simulink model "testStateflow"  (R2014a)
settings: Solver=FixedStepDiscrete  StartTime=0.0  StopTime=Inf  FixedStep=0.001  RelTol=1e-3
settings Model: BufferReuse=off  Creator=djoshea  LastModifiedBy=djoshea
settings SolverCC: EnableConcurrentExecution=on
settings OptimizationCC: BlockReduction=off  OptimizeBlockIOStorage=off  BufferReuse=off  GlobalBufferReuse=off  ExpressionFolding=off  LocalBlockOutputs=off
settings HardwareCC: ProdIntDivRoundTo=Zero  ProdEndianess=LittleEndian  ProdHWDeviceType=Generic->32-bit x86 compatible
settings RTWCC: SystemTargetFile=slrt.tlc  TemplateMakefile=slrt_default_tmf  Description=Simulink Real-Time  ProcessScript=slrt_make_rtw_hook  RTWCompilerOptimization=On
settings SimulinkRealTimeCC: GeneratePreprocessorConditionals=Disable all  EnableShiftOperators=on

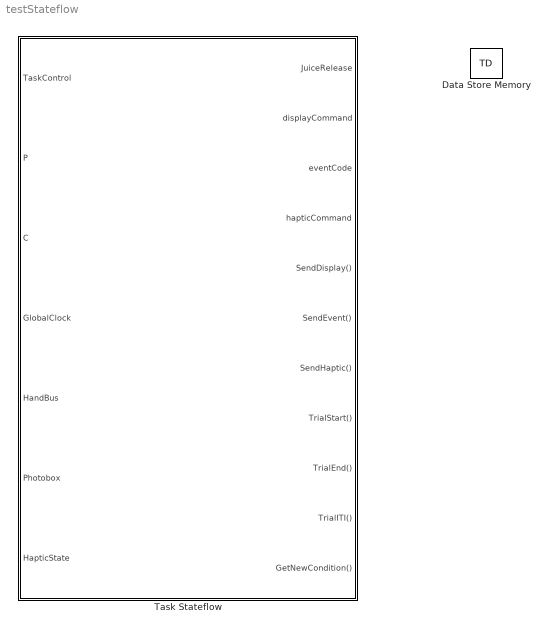
== system testStateflow ==
  Data Store Memory : DataStoreMemory  DataStoreName=TD  ReadBeforeWriteMsg=warning  WriteAfterWriteMsg=warning  WriteAfterReadMsg=warning  OutDataTypeStr=Bus: TrialDataBus
  Task Stateflow : Stateflow chart  TreatAsAtomicUnit=on

== stateflow chart testStateflow/Task Stateflow ==
  state TaskControl [parallel]
    settings: executionOrder=1
    state Task
      state TaskFlow [parallel]
        ex:
        send(HapticReset, HapticMoveHoldControl);
        send(HapticDisallowPerturbation, HapticPerturbationControl);
        send(AbortJuice, JuiceToggle);
        settings: executionOrder=1
        state InitTrial
          en:
          send(TrialStart);
          TD.taskRunning = uint8(1);
          displayCommand = DisplayCommand.InitTrial;
          send(SendDisplay);
          hapticCommand = HapticCommand.SupportAtCenter;
          send(SendHaptic);
          send(HapticAllowPerturbation, HapticPerturbationControl);
          eventCode = TaskEvent.CenterOnset;
          state = TaskState.InitTrial;
          TD.timeInitTrial = GlobalClock;
          TD.timeGoCueCommand = uint32(0);
          TD.timeGoCue = uint32(0);
          TD.timeTargetOnsetCommand = uint32(0);
          TD.timeTargetOnset = uint32(0);
          TD.timeMove = uint32(0);
          TD.rt = uint32(0);
          TD.rtNominal = uint32(0);
          TD.delay = uint32(0);
          TD.iti = uint32(0);
          TD.holdXCenter = 0;
          TD.holdYCenter = 0;
          TD.holdXTarget = 0;
          TD.holdYTarget = 0;
          TD.targetXCurrent = 0;
          TD.targetYCurrent = 0;
          TD.targetWidthCurrent = 0;
          TD.targetDepthCurrent = 0;
          TD.hapticPerturbationOccurred = uint8(0);
          TD.hitObstacleThisTrial = uint8(0);
          TD.consecutiveNoStarts = TD.consecutiveNoStarts + uint16(1);
          TD.isTouchingTarget = uint8(0);
          TD.hasMissedTarget = uint8(0);
          TD.substantiveFailure = uint8(0);
          TD.moveOnsetThreshOccurred = uint8(0);
        state CenterAcquireHold
          state CenterAcquireLogic [parallel]
            settings: executionOrder=1
            state WaitCenterSettle
              en:
              state = TaskState.WaitCenterSettle;
              displayCommand = DisplayCommand.CenterAcquired;
              send(SendDisplay);
              eventCode = TaskEvent.CenterAcquired;
              send(SendEvent);
              ex:
              % Establish hold window for td.isHolding
              TD.holdXCenter = HandBus.handX;
              TD.holdYCenter = HandBus.handY;
            state WaitCenterAcquire
              en:
              state = TaskState.WaitCenterAcquire;
              displayCommand = DisplayCommand.CenterOnset;
              send(SendDisplay);
              eventCode = TaskEvent.CenterOnset;
              send(SendEvent);
              % Move the hand to the center (while he's holding on)
              send(HapticMoveToCenter, HapticMoveHoldControl);
            state WaitCenterHold
              en:
              state = TaskState.WaitCenterHold;
              displayCommand = DisplayCommand.CenterSettled;
              send(SendDisplay);
              eventCode = TaskEvent.CenterSettled;
              send(SendEvent);
              % Either stop moving to center or hold the haptic for the delay period
              send(HapticArrivedAtCenter, HapticMoveHoldControl);
            state CenterUnacquire
              en:
              displayCommand = DisplayCommand.CenterUnacquire;
              send(SendDisplay);
              eventCode = TaskEvent.CenterUnacquire;
              send(SendEvent);
            state CenterHeld
              en:
              displayCommand = DisplayCommand.CenterHeld;
              send(SendDisplay);
              eventCode = TaskEvent.CenterHeld;
              send(SendEvent);
              % always send target to haptic, command packet will indicate
              % whether viscosity is needed
              hapticCommand = HapticCommand.CreateTarget;
              send(SendHaptic);
              if P.timeJuiceCenter > 0
              TD.juiceNumDrops = uint16(1);
              TD.juiceDropSize = uint16(P.timeJuiceCenter);
              send(SendJuice, JuiceToggle);
              end
            WaitCenterAcquire -> WaitCenterSettle [order 1] : [TD.isTouchingCenter == 1]
            CenterUnacquire -> WaitCenterAcquire
            WaitCenterSettle -> WaitCenterHold : after(P.timeCenterSettle,tick)
                | % Wait for settling before enforcing hold
            WaitCenterHold -> CenterUnacquire [order 3] : [~TD.isHoldingCenter && P.allowReacquireCenter]
                | % Moved during center hold --> allow re-aquire
            WaitCenterHold -> CenterHeld [order 2] : after(P.timeCenterHold,tick)
                | % Held center
        state StartTask
          en:
          state = TaskState.StartTask;
          displayCommand = DisplayCommand.StartTask;
          send(SendDisplay);
        state GetNewTrialParams
          en:
          send(GetNewCondition);
        state HoldingHaptic
          state DelayPeriodGoCue
            state ShowObstacle
              en:
              hapticCommand = HapticCommand.CreateGap;
              send(SendHaptic);
              displayCommand = DisplayCommand.ObstacleOnset;
              send(SendDisplay);
              eventCode = TaskEvent.ObstacleOnset;
              send(SendEvent);
            state GoCue
              en:
              send(HapticGoCue, HapticMoveHoldControl);
              state GoCueZeroDelay
                en:
                state = TaskState.GoCueZeroDelay;
                TD.timeGoCueCommand = GlobalClock;
                displayCommand = DisplayCommand.GoCueZeroDelay;
                send(SendDisplay);
                eventCode = TaskEvent.TargetOnsetCommand;
                send(SendEvent);
                eventCode = TaskEvent.GoCueCommand;
                send(SendEvent);
              state GoCueNonZeroDelay
                en:
                state = TaskState.GoCueNonZeroDelay;
                TD.timeGoCueCommand = GlobalClock;
                displayCommand = DisplayCommand.GoCueNonZeroDelay;
                send(SendDisplay);
                eventCode = TaskEvent.GoCueCommand;
                send(SendEvent);
            state SetTargetInfo
              en:
              TD.targetXCurrent = C.targetX;
              TD.targetYCurrent = C.targetY;
              TD.targetWidthCurrent = C.targetWidth;
              TD.targetDepthCurrent = C.targetDepth;
            state DelayPeriod
              en:
              state = TaskState.DelayPeriod;
              TD.timeTargetOnsetCommand = GlobalClock;
              displayCommand = DisplayCommand.DelayPeriodStart;
              send(SendDisplay);
              eventCode = TaskEvent.TargetOnsetCommand;
              send(SendEvent);
            state WaitMoveOnset
              en:
              state = TaskState.WaitMoveOnset;
              du:
              TD.rt = GlobalClock - TD.timeGoCue; % detected by photobox
              TD.rtNominal = GlobalClock - TD.timeGoCueCommand; % not detected by photobox
              ex:
              TD.timeMove = GlobalClock;
              TD.rt = GlobalClock - TD.timeGoCue; % not detected by photobox
              TD.rtNominal = GlobalClock - TD.timeGoCueCommand; % not detected by photobox
              send(HapticMoveOnset, HapticMoveHoldControl);
              displayCommand = DisplayCommand.MoveOnset;
              send(SendDisplay)
              eventCode = TaskEvent.MoveOnsetOnline;
              send(SendEvent);
            (default) -> (junction 1909)
            (junction 1909) -> ShowObstacle [order 1] : [C.hasChannel]
            (junction 1909) -> SetTargetInfo [order 2]
            ShowObstacle -> (junction 1923) [order 2] : [~TD.isHoldingCenter]
                | % Moved during delay
            ShowObstacle -> SetTargetInfo [order 1] : % Show obstacle first, then target
                | after(C.timeObstacleOnsetBeforeTarget, tick)
            SetTargetInfo -> GoCueZeroDelay [order 1] : [C.delayNominal == 0]
                | % Zero Delay
            DelayPeriod -> (junction 1923) [order 1] : [~TD.isHoldingCenter]
                | % Moved during delay
            SetTargetInfo -> DelayPeriod [order 2] : % Non-zero Delay
            DelayPeriod -> GoCueNonZeroDelay [order 2] : after(C.delayNominal, tick)
                | % Delay period over
            GoCue -> WaitMoveOnset : after(1,tick)
            WaitMoveOnset -> (junction 1269) [order 2] : [~TD.isHoldingCenter]
                | % Move from center
          state TargetAcquireHold
            state WaitTargetAcquire
              en:
              TD.consecutiveNoStarts = uint16(0); % count as initiated the trial
              state = TaskState.WaitTargetAcquire;
            state WaitTargetHold
              en:
              send(HapticHoldAtTarget, HapticMoveHoldControl);
              TD.holdXTarget = HandBus.handX;
              TD.holdYTarget = HandBus.handY;
              state = TaskState.WaitTargetHold;
              displayCommand = DisplayCommand.TargetSettled;
              send(SendDisplay);
              eventCode = TaskEvent.TargetSettled;
              send(SendEvent);
              ex:
              displayCommand = DisplayCommand.TargetHeld;
              send(SendDisplay);
              eventCode = TaskEvent.TargetHeld;
              send(SendEvent);
            WaitTargetAcquire -> WaitTargetHold [order 2] : [TD.isTouchingTarget || currentlyTouching]
                | % Target Acquired
          (junction 1269) -> WaitTargetAcquire [order 1] : [TD.rtNominal >= P.rtMin]
              | % RT acceptable
        state TrialFailure
          en:
          TD.success = uint8(0);
          send(HapticDisallowPerturbation, HapticPerturbationControl);
          state FailureCenterAcquire
            en:
            TD.substantiveFailure = uint8(0);
            state = TaskState.FailureCenterAcquire;
            TD.getNewTrialParams = uint8(0);
            displayCommand = DisplayCommand.FailureCenterFlyAway;
            send(SendDisplay);
            eventCode = TaskEvent.FailureToAcquireCenter;
            send(SendEvent);
          state FailureComputeITI
            en:
            if P.repeatUntilSuccess
            TD.getNewTrialParams = uint8(0);
            end
            TD.failureCode = state;
            computeFailureITI();
          state FailureHitObstacle
            en:
            state = TaskState.FailureHitObstacle;
            TD.getNewTrialParams = uint8(1);
            TD.substantiveFailure = uint8(1);
            displayCommand = DisplayCommand.FailureHitObstacle;
            send(SendDisplay);
            eventCode = TaskEvent.FailureHitObstacle;
            send(SendEvent);
          state FailureClearObstacles
            en:
            hapticCommand = HapticCommand.ClearObstacles;
            send(SendHaptic);
          state FailureCenterHold
            en:
            TD.substantiveFailure = uint8(0);
            state = TaskState.FailureCenterHold;
            TD.getNewTrialParams = uint8(0);
            displayCommand = DisplayCommand.FailureCenterFlyAway;
            send(SendDisplay);
            eventCode = TaskEvent.FailureBrokeCenterHold;
            send(SendEvent);
          state FailureDelayMove
            en:
            TD.substantiveFailure = uint8(0);
            state = TaskState.FailureDelayMove;
            TD.getNewTrialParams = uint8(1);
            displayCommand = DisplayCommand.FailureTargetFlyAway;
            send(SendDisplay);
            eventCode = TaskEvent.FailureBrokeCenterHoldDelay;
            send(SendEvent);
          state FailureRTTooFast
            en:
            TD.substantiveFailure = uint8(0);
            state = TaskState.FailureRTTooFast;
            TD.getNewTrialParams = uint8(0);
            displayCommand = DisplayCommand.FailureTargetFlyAway;
            send(SendDisplay);
            eventCode = TaskEvent.FailureRTTooFast;
            send(SendEvent);
          state FailureRTTooSlow
            en:
            TD.substantiveFailure = uint8(0);
            state = TaskState.FailureRTTooSlow;
            TD.getNewTrialParams = uint8(0);
            displayCommand = DisplayCommand.FailureTargetFlyAway;
            send(SendDisplay);
            eventCode = TaskEvent.FailureRTTooSlow;
            send(SendEvent);
          state FailureMissedTarget
            en:
            TD.substantiveFailure = uint8(1);
            state = TaskState.FailureTargetMissed;
            TD.getNewTrialParams = uint8(1);
            displayCommand = DisplayCommand.FailureTargetFlyAway;
            send(SendDisplay);
            eventCode = TaskEvent.MissedTarget;
            send(SendEvent);
            eventCode = TaskEvent.FailureTargetMissed;
            send(SendEvent);
          state FailureTargetAcquire
            en:
            TD.substantiveFailure = uint8(1);
            state = TaskState.FailureTargetAcquire;
            TD.getNewTrialParams = uint8(1);
            displayCommand = DisplayCommand.FailureTargetFlyAway;
            send(SendDisplay);
            eventCode = TaskEvent.FailureToAcquireTarget;
            send(SendEvent);
          state FailureHapticReleased
            en:
            TD.substantiveFailure = uint8(0);
            state = TaskState.FailureHapticReleased;
            TD.getNewTrialParams = uint8(1);
            displayCommand = DisplayCommand.FailureTargetFlyAway;
            send(SendDisplay);
            eventCode = TaskEvent.FailureHapticReleased;
            send(SendEvent);
          FailureCenterAcquire -> (junction 1353)
          FailureHitObstacle -> (junction 1857) : % Bypass obstacle clearing when hit
          (junction 1857) -> FailureComputeITI
          FailureClearObstacles -> (junction 1857)
          (junction 1353) -> FailureClearObstacles : after(1,tick)
          FailureCenterHold -> (junction 1353)
          FailureHapticReleased -> (junction 1353)
          FailureDelayMove -> (junction 1353)
          FailureRTTooFast -> (junction 1353)
          FailureTargetAcquire -> (junction 1353)
          FailureRTTooSlow -> (junction 1353)
          FailureMissedTarget -> (junction 1353)
        state ITI
          en:
          send(TrialEnd);
          state = TaskState.ITI;
          displayCommand = DisplayCommand.ITI;
          send(SendDisplay);
          send(TrialITI);
          % Reset the haptic to normal state
          send(HapticReset, HapticMoveHoldControl);
          send(HapticDisallowPerturbation, HapticPerturbationControl);
        state Success
          en:
          state = TaskState.Success;
          TD.success = uint8(1);
          TD.getNewTrialParams = uint8(1);
          computeRewardAndITI();
          send(SendJuice, JuiceToggle);
          displayCommand = DisplayCommand .Success;
          send(SendDisplay);
          eventCode = TaskEvent.Success;
          send(SendEvent);
        (default) -> StartTask
        GetNewTrialParams -> InitTrial : after(1, tick)
        (junction 1387) -> InitTrial [order 2] : % Re-use the old trial params
        StartTask -> GetNewTrialParams : after(1,tick)
        (junction 1387) -> GetNewTrialParams [order 1] : [TD.getNewTrialParams>0]
            | % New condition needed
        ITI -> (junction 1387) : after(TD.iti,tick)
            | % Wait ITI
        Success -> ITI : after(P.timeRewardFeedback,tick)
            | % Wait for target white flash
        WaitTargetAcquire -> FailureMissedTarget [order 3] : % Went past planar stop target
            | [TD.hasMissedTarget && P.failOnMissedTarget]
        FailureComputeITI -> ITI : after(TD.timeFailureFeedback,tick)
        WaitCenterAcquire -> FailureCenterAcquire [order 2] : after(P.timeCenterAcquire,tick)
            | % Did not acquire center
        WaitCenterHold -> FailureCenterHold [order 1] : [~TD.isHoldingCenter && ~P.allowReacquireCenter]
            | % Moved during center hold --> fail trial
        (junction 1923) -> CenterUnacquire [order 2] : [P.allowReacquireCenter]
            | % Moved during delay --> allow-reacquire
        WaitTargetAcquire -> FailureTargetAcquire [order 1] : after(P.timeTargetAcquire, tick)
            | % Did not acquire target
        InitTrial -> WaitCenterAcquire : after(1,tick)
        (junction 1923) -> FailureDelayMove [order 1] : [~P.allowReacquireCenter]
            | % Moved during delay -> fail trial
        CenterHeld -> DelayPeriodGoCue
        WaitTargetHold -> Success : after(P.timeTargetHold, tick)
            | % Held target
        HoldingHaptic -> FailureHitObstacle [order 2] : [HapticState.hitObstacle && ...
            | (~C.obstacleCollisionPermitted)]
            | % Hit red obstacle
        (junction 1269) -> FailureRTTooFast [order 2] : [TD.rtNominal < P.rtMin]
            | % RT too fast
        WaitMoveOnset -> FailureRTTooSlow [order 1] : after(P.rtMax,tick)
            | % RT too slow
        HoldingHaptic -> FailureHapticReleased [order 1] : [~HandBus.handSeen]
            | % Released haptic device
      state HapticObstacleState [parallel]
        settings: executionOrder=6
        state DebounceRelease
        state NotColliding
        state DebounceHit
        state Colliding
          en:
          TD.hitObstacleThisTrial = uint8(1);
          displayCommand = DisplayCommand.HitObstacle;
          send(SendDisplay);
          eventCode = TaskEvent.HitObstacle;
          send(SendEvent);
          ex:
          displayCommand = DisplayCommand.ReleasedObstacle;
          send(SendDisplay);
          eventCode = TaskEvent.ReleasedObstacle;
          send(SendEvent);
        (default) -> NotColliding
        DebounceRelease -> DebounceHit [order 1] : [HapticState.hitObstacle == 1]
        DebounceRelease -> NotColliding [order 2] : after(100, tick)
        DebounceHit -> DebounceRelease : [HapticState.hitObstacle==0]
        Colliding -> DebounceRelease : [HapticState.hitObstacle==0]
        NotColliding -> Colliding : [HapticState.hitObstacle == 1]
      state ComputeHandState [parallel]
        en,du:
        if state ~= TaskState.InitTrial
        % determine if we're within the center hold windows
        TD.isTouchingCenter = isTouching(C.centerX, C.centerY, P.centerSize);
        TD.isHoldingCenter = uint8(isTouching(TD.holdXCenter, TD.holdYCenter, P.holdWindowCenter) && ~HandBus.handMoving);
        % always use haptic coordinates to determine touching
        % if hand passes vertically above target without colliding, register a miss
        currentlyTouching = uint8(0);
        currentlyPastTarget = uint8(0);
        [currentlyTouching, currentlyPastTarget] = isTouchingBarTarget();
        if ~TD.hasMissedTarget && currentlyTouching && TD.timeTargetOnsetCommand > 0
        % mark target as touched
        TD.isTouchingTarget = uint8(1);
        end
        if ~TD.isTouchingTarget && ~TD.hasMissedTarget && currentlyPastTarget && TD.timeTargetOnsetCommand > 0
        % mark target as missed
        TD.hasMissedTarget = uint8(1);
        end
        if TD.timeGoCueCommand > 0
        % figure out our distance/velocity in direction of target
        [TD.distanceTowardsTarget, TD.velocityTowardsTarget] = computeProgressTowardsTarget();
        if ~TD.moveOnsetThreshOccurred && ...
        TD.velocityTowardsTarget >= P.velocityTowardsTargetThresh && ...
        TD.distanceTowardsTarget >= P.distanceTowardsTargetThresh
        TD.moveOnsetThreshOccurred = uint8(1);
        eventCode = TaskEvent.MoveOnsetThresh;
        send(SendEvent);
        end
        end
        end
        settings: executionOrder=2
      state PhotoboxEvents [parallel]
        settings: executionOrder=3
        state PhotoboxOnZeroDelayTrial
          en:
          eventCode = TaskEvent.TargetOnset;
          TD.timeTargetOnset = GlobalClock;
          send(SendEvent);
        state PhotoboxSendGoCue
          en:
          eventCode = TaskEvent.GoCue;
          TD.timeGoCue = GlobalClock;
          TD.delay = TD.timeGoCue - TD.timeTargetOnset;
          send(SendEvent);
        state PhotoboxOnDelayTrial
          en:
          eventCode = TaskEvent.TargetOnset;
          TD.timeTargetOnset = GlobalClock;
          send(SendEvent);
        state PhotoboxOff
        PhotoboxOnZeroDelayTrial -> PhotoboxSendGoCue
        PhotoboxOnDelayTrial -> PhotoboxSendGoCue : [Photobox==0]
        (junction 1713) -> PhotoboxOnZeroDelayTrial [order 2] : [C.delayNominal == 0]
        PhotoboxSendGoCue -> PhotoboxOff : [Photobox==0]
        (default) -> PhotoboxOff
        (junction 1713) -> PhotoboxOnDelayTrial [order 1] : [C.delayNominal > 0]
        PhotoboxOff -> (junction 1713) : [Photobox==1]
      state HapticMoveHoldControl [parallel]
        settings: executionOrder=5
        state NotSeenFreeze
          en:
          hapticCommand = HapticCommand.MoveToHoldNotSeen;
          send(SendHaptic);
        state HapticReset
          en:
          hapticCommand = HapticCommand.ClearObstacles;
          send(SendHaptic);
          hapticCommand = HapticCommand.ClearTarget;
          send(SendHaptic);
        state HapticMoveToCenterWhileHandSeen
          state WaitHandleTouch
            en:
            hapticCommand = HapticCommand.MoveToHoldNotSeen;
            send(SendHaptic);
          state WaitHandleHeld
            % Debouncing for handSeen
          state HandleHeld
            en:
            hapticCommand = HapticCommand.MoveToCenter;
            send(SendHaptic);
          WaitHandleTouch -> WaitHandleHeld : [HandBus.handSeen]
          WaitHandleHeld -> WaitHandleTouch [order 1] : [~HandBus.handSeen]
          (default) -> WaitHandleTouch [order 2]
          HandleHeld -> WaitHandleTouch : [~HandBus.handSeen]
          WaitHandleHeld -> HandleHeld [order 2] : after(300,tick)
          (default) -> HandleHeld [order 1] : [HandBus.handSeen]
        state HapticInTask
          state HapticHoldAtTarget
            en:
            hapticCommand = HapticCommand.ConstrainToPoint;
            send(SendHaptic);
            ex:
            hapticCommand = HapticCommand.ConstrainAbort;
            send(SendHaptic);
          state HapticMoveOnset
          state HapticGoCue
          state HapticArrivedAtCenter
            state HapticHoldDuringDelay
              % Move to center remains active until go cue
              ex:
              hapticCommand = HapticCommand.MoveAbort;
              send(SendHaptic);
            state HapticReleaseDuringDelay
              en:
              hapticCommand = HapticCommand.MoveAbort;
              send(SendHaptic);
            (default) -> HapticHoldDuringDelay [order 1] : [P.manualHoldDuringDelay == 1]
            (default) -> HapticReleaseDuringDelay [order 2]
          HapticMoveOnset -> HapticHoldAtTarget : HapticHoldAtTarget
          HapticGoCue -> HapticMoveOnset : HapticMoveOnset
          HapticArrivedAtCenter -> HapticGoCue [order 1] : HapticGoCue
        NotSeenFreeze -> HapticReset [order 1] : HapticReset
        NotSeenFreeze -> HapticMoveToCenterWhileHandSeen [order 2] : HapticMoveToCenter
        (default) -> HapticReset
        HapticReset -> NotSeenFreeze [order 1] : [~HandBus.handSeen]
        HapticReset -> HapticMoveToCenterWhileHandSeen [order 2] : HapticMoveToCenter
        HapticInTask -> HapticReset [order 1] : HapticReset
        HapticInTask -> NotSeenFreeze [order 2] : [~HandBus.handSeen]
        HapticArrivedAtCenter -> HapticMoveToCenterWhileHandSeen [order 2] : HapticMoveToCenter
        HapticMoveToCenterWhileHandSeen -> HapticArrivedAtCenter : HapticArrivedAtCenter
      state JuiceToggle [parallel]
        settings: executionOrder=4
        state JuiceDeliverDrops
          en:
          TD.juiceDropsRemaining = TD.juiceNumDrops;
          ex:
          JuiceRelease = uint8(0);
          state JuiceDropInterval
            en:
            JuiceRelease = uint8(0);
            TD.juiceDropsRemaining = TD.juiceDropsRemaining - uint16(1);
          state JuiceDropReleasing
            en:
            JuiceRelease  = uint8(1);
          (default) -> JuiceDropReleasing
          JuiceDropReleasing -> JuiceDropInterval : after(TD.juiceDropSize, tick)
          JuiceDropInterval -> JuiceDropReleasing [order 2] : after(TD.juiceDropInterval - TD.juiceDropSize, tick)
        state Off
          en:
          JuiceRelease = uint8(0);
        Off -> JuiceDropReleasing : SendJuice
        JuiceDropInterval -> Off [order 1] : [TD.juiceDropsRemaining < 1 || TD.juiceDropsRemaining > 10]
        JuiceDeliverDrops -> Off : AbortJuice
        (default) -> Off
      state HapticPerturbationControl [parallel]
        settings: executionOrder=7
        state HapticAllowPerturbMode
          state HapticWaitPerturb
          state HapticSendPerturb
            en:
            TD.hapticPerturbationOccurred = uint8(1);
            hapticCommand = HapticCommand.PulsePerturbation;
            send(SendHaptic);
            eventCode = TaskEvent.HapticPerturbation;
            send(SendEvent);
            eventCode = TaskEvent.HapticPerturbationOption;
            send(SendEvent);
            % shift target
            if C.targetShiftPostPerturbation
            displayCommand = DisplayCommand.TargetShift;
            send(SendDisplay);
            eventCode = TaskEvent.TargetShift;
            send(SendEvent);
            TD.targetXCurrent = C.targetXPostShift;
            TD.targetYCurrent = C.targetYPostShift;
            TD.targetWidthCurrent = C.targetWidthPostShift;
            TD.targetDepthCurrent = C.targetDepthPostShift;
            end
          state WaitEventOffset
          state ShamPerturbation
            en:
            eventCode = TaskEvent.HapticPerturbationOption;
            send(SendEvent);
          state ShamPerturbationEnd
            en:
            eventCode = TaskEvent.HapticPerturbationOptionEnd;
            send(SendEvent);
          state HapticPerturbEnd
            en:
            eventCode = TaskEvent.HapticPerturbationEnd;
            send(SendEvent);
            eventCode = TaskEvent.HapticPerturbationOptionEnd;
            send(SendEvent);
          (default) -> HapticWaitPerturb
          HapticWaitPerturb -> WaitEventOffset : % Perturbation-locked event
              | [eventCode == C.perturbRelativeToEvent]
          WaitEventOffset -> (junction 2065) : after(C.perturbOffsetFromEvent, tick)
          (junction 2065) -> HapticSendPerturb [order 1] : [C.perturb]
          (junction 2065) -> ShamPerturbation [order 2] : [~C.perturb] % fake perturbation for event alignment purposes
          ShamPerturbation -> ShamPerturbationEnd : after(C.perturbDuration, tick)
          HapticSendPerturb -> HapticPerturbEnd : after(C.perturbDuration, tick)
        state HapticAbortLetGo
          en:
          hapticCommand = HapticCommand.PerturbationAbort;
          send(SendHaptic);
        state HapticDisallowPerturbMode
          en:
          hapticCommand = HapticCommand.PerturbationAbort;
          send(SendHaptic);
        ShamPerturbationEnd -> HapticDisallowPerturbMode
        HapticPerturbEnd -> HapticDisallowPerturbMode
        HapticDisallowPerturbMode -> HapticAllowPerturbMode : HapticAllowPerturbation
        HapticAllowPerturbMode -> HapticDisallowPerturbMode [order 2] : HapticDisallowPerturbation
        HapticAllowPerturbMode -> HapticAbortLetGo [order 1] : [HandBus.handSeen == 0]
        (junction 2019) -> HapticAllowPerturbMode : % Debouncing
            | after(30, tick)
        HapticAbortLetGo -> (junction 2019) : [HandBus.handSeen == 1]
        (default) -> HapticDisallowPerturbMode
  data: tf function_output uint8 size=1; boxX function_input double; boxY function_input double; boxSize function_input double; tfTouching function_output uint8 size=1; tfMissed function_output uint8 size=1; distance function_output double size=1; velocity function_output double size=1; currentlyPastTarget local uint8 size=1; currentlyTouching local uint8 size=1; JuiceRelease output uint8 size=1; TaskControl input Bus: TaskControlBus size=1; P input Bus: ParamBus size=1; state local Enum: TaskState size=1; C input Bus: ConditionBus size=1; GlobalClock input uint32 size=1; displayCommand output Enum: DisplayCommand size=1; HandBus input Bus: HandBus size=1; Photobox input size=1; TD data_store_memory; eventCode output Enum: TaskEvent size=1; hapticCommand output Enum: HapticCommand size=1; HapticState input Bus: HapticInputBus size=1
  events: HapticMoveToCenter local FUNCTION_CALL_EVENT; AbortJuice local FUNCTION_CALL_EVENT; HapticMoveOnset local FUNCTION_CALL_EVENT; HapticGoCue local FUNCTION_CALL_EVENT; HapticArrivedAtCenter local FUNCTION_CALL_EVENT; HapticHoldAtTarget local FUNCTION_CALL_EVENT; HapticReset local FUNCTION_CALL_EVENT; HapticAllowPerturbation local FUNCTION_CALL_EVENT; HapticDisallowPerturbation local FUNCTION_CALL_EVENT; SendJuice local FUNCTION_CALL_EVENT; SendDisplay output FUNCTION_CALL_EVENT; SendEvent output FUNCTION_CALL_EVENT; SendHaptic output FUNCTION_CALL_EVENT; TrialStart output FUNCTION_CALL_EVENT; TrialEnd output FUNCTION_CALL_EVENT; TrialITI output FUNCTION_CALL_EVENT; GetNewCondition output FUNCTION_CALL_EVENT
  function tf = isTouching(boxX, boxY, boxSize):
    | function tf = isTouching(boxX, boxY, boxSize)
    | 
    | x = HandBus.handX;
    | y = HandBus.handY;
    | z = HandBus.handZ;
    | 
    | if HandBus.handSeen && HandBus.handTouching && ...
    |    abs(x - boxX) < boxSize/2 && ...
    |    abs(y - boxY) < boxSize/2
    | 
    |     tf = uint8(1);
    | else
    |     tf = uint8(0);
    | end
  function [tfTouching, tfMissed] = isTouchingBarTarget:
    | function [tfTouching, tfMissed] = isTouchingBarTarget
    | % given the Condition and hand position, compute whether
    | % the hand is in the target. Score is a double that ranges from 0 to 1, 
    | % which will indicate some metric of lateral deviation
    | 
    | hx = HandBus.handX;
    | hy = HandBus.handY;
    | tx = C.targetXPostShift;
    | ty = C.targetYPostShift;
    | width = C.targetWidthPostShift;
    | depth = C.targetDepthPostShift;
    | 
    | % translate/rotate target and hand coordinates so that target rectangle is at 
    | % X: -width/2 to +width/2
    | % Y: -depth/2 to +depth/2
    | thetaOrientation = C.targetTheta;
    | rot = [ cos(thetaOrientation), sin(thetaOrientation); ...
    |        -sin(thetaOrientation), cos(thetaOrientation)];
    | rotHand = rot * [hx - tx; hy - ty];
    | rhx = rotHand(1);
    | rhy = rotHand(2);
    | 
    | % targXMin = -depth/2;
    | % targXMax = +depth/2;
    | % targYMin = -width/2;
    | % targYMax =  width/2;
    | 
    | targXMin = -width/2 - P.hapticCursorDiameter/2;
    | targXMax =  width/2 + P.hapticCursorDiameter/2;
    | targYMin = -depth/2 - P.hapticCursorDiameter/2;
    | targYMax = +depth/2 + P.hapticCursorDiameter/2;
    | 
    | if HandBus.handSeen && HandBus.handTouching && ...
    |    rhx >= targXMin && rhx <= targXMax && ...
    |    rhy >= targYMin
    |    
    |     % inside the bar
    |     tfTouching = uint8(1);
    |     tfMissed = uint8(0);
    | elseif HandBus.handSeen && HandBus.handTouching && ...
    |    (rhx < targXMin || rhx > targXMax) && ... % outside the target in X
    |    (rhy >= targYMin + P.handMissedTargetMargin)
    |    
    |     % missed the bar
    |     tfMissed = uint8(1);
    |     tfTouching = uint8(0);
    |     
    | else
    |     
    |     % neither yet
    |     tfTouching = uint8(0);
    |     tfMissed = uint8(0);
    | end
  function [distance, velocity] = computeProgressTowardsTarget:
    | function [distance, velocity] = computeProgressTowardsTarget()
    | % given the Condition and hand position, compute whether
    | % the hand is in the target. Score is a double that ranges from 0 to 1, 
    | % which will indicate some metric of lateral deviation
    | 
    | hx = HandBus.handX;
    | hy = HandBus.handY;
    | vx = HandBus.handVelocityX;
    | vy = HandBus.handVelocityY;
    | cx = C.centerX;
    | cy = C.centerY;
    | width = TD.targetWidthCurrent;
    | depth = TD.targetDepthCurrent;
    | 
    | % translate/rotate target and hand coordinates so that target is straight upwards, i.e. at
    | % X: -width/2 to +width/2
    | % Y: targetDistance +/- targetDepth/2
    | thetaOrientation = C.targetTheta;
    | rot = [ cos(thetaOrientation), sin(thetaOrientation); ...
    |        -sin(thetaOrientation), cos(thetaOrientation)];
    | rotHand = rot * [hx - cx; hy - cy];
    | rhx = rotHand(1);
    | rhy = rotHand(2);
    | rotVel =  rot * [vx; vy];
    | rvx = rotVel(1);
    | rvy = rotVel(2);
    | 
    | distance = 0;
    | velocity = 0;
    | 
    | if HandBus.handSeen && HandBus.handTouching
    |     distance = rhy;
    |     velocity = rvy;
    | end
  function computeFailureITI:
    | function computeFailureITI()
    | 
    | TD.timeFailureFeedback = P.timeFailureFeedback;
    | TD.iti = P.itiFailure;
    | TD.juiceTimeTotal = uint32(0);
    | 
    | %if TD.failureCode == State.FailureHitObstacle
    | %    TD.iti = uint32(0);
    | %else
    | %    TD.timeFailureFeedbac%k = uint32(1);
    | %end
  function computeRewardAndITI:
    | function computeRewardAndITI()
    | % split juice into discrete drops and compute the pulse train to play as
    | % the reward signal
    | 
    | TD.juiceTimeTotal = uint32(P.timeJuice); 
    | %if TD.hitObstacleThisTrial
    |     % halve the reward following obstacle collisions
    | %    TD.juiceTimeTotal = uint32(P.timeJuiceHitObstacle);
    | %end
    | 
    | TD.juiceNumDrops = uint16(1);
    | TD.juiceDropSize = uint16(TD.juiceTimeTotal);
    | 
    | TD.juiceDropInterval = uint16(400);
    | 
    | % 20140409 separating tone from reward size since reward size carries
    | % no information now
    | %TD.rewardTonePulseHz = TD.targetAccuracyScore * freqMultiplier + minFreq;
    | TD.rewardTonePulseHz = 2200;
    | TD.rewardTonePulseLength = uint16(200);
    | TD.rewardTonePulseInterval = TD.juiceDropInterval;
    | %TD.rewardTonePulseReps = TD.juiceNumDrops;
    | TD.rewardTonePulseReps = uint16(3);
    | 
    | if TD.hitObstacleThisTrial
    |     TD.iti = P.itiFailure;
    | else
    |     TD.iti = P.itiSuccess;
    | end 
    | 
    | end
